simulink model "PID_control"  (R2020b)
settings: Solver=VariableStepAuto  StartTime=0.0  StopTime=10.0  RelTol=1e-3
model workspace (MAT data in the model file):
  J = 3.2284e-06
  K = 0.0274
  L = 2.75e-06
  R = 4
  b = 3.5077e-06
  kd = 0.139068731322
  ki = 523.29550805
  kp = 17.36824987
settings Model: Creator=com  LastModifiedBy=com
settings DataIOCC: SaveOutput=off  SaveTime=off

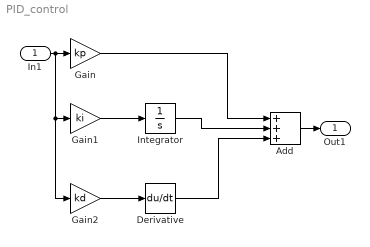
== system PID_control ==
  In1 : Inport  OutDataTypeStr=double  PortDimensions=1
  Add : Sum  Inputs=+++
  Derivative : Derivative
  Gain : Gain  Gain=kp
  Gain1 : Gain  Gain=ki
  Gain2 : Gain  Gain=kd
  Integrator : Integrator
  Out1 : Outport  OutDataTypeStr=double  PortDimensions=1  SampleTime=0
  wires:
  Gain1/1 -> Integrator/1
  Gain/1 -> Add/1
  Derivative/1 -> Add/3
  Integrator/1 -> Add/2
  Add/1 -> Out1/1
  Gain2/1 -> Derivative/1
  In1/1 -> Gain/1, Gain1/1, Gain2/1
